simulink model "RobotArm_ForwardDynamics"  (R2024b)
settings: Solver=FixedStepAuto  StartTime=0.0  StopTime=5  FixedStep=1e-4  MaxStep=1e-4  RelTol=1e-3
InitFcn:
  | % Working Directory
  | % currDir = pwd;
  | % Import results from HoG
  | load('refAngles_HoG.mat')
  | 
  | data = thetas';
  | refA  = data(:,[1  2]);
  | refBE = data(:,[1  3]);
  | refBD = data(:,[1  4]);
  | refG  = data(:,[1  8]);
  | refH  = data(:,[1  9]);
  | refI  = data(:,[1 10]);
model workspace (MATLAB code in the model file):
  | %% General Parameters
  | 
  | g = 9.81; % [m/sec^2] assuming we are on earth :)
  | 
  | %% Chosen Parameters
  | 
  | % Gearbox Ratios
  | iA  = 20;
  | iBE = 20;
  | iBD = 20;
  | iG  = 20;
  | iH  = 20;
  | iI  = 20;
  | 
  | % Servomotor Torque Constants
  | KmA  = 0.5; % [Nm/A]
  | KmBE = 0.5; % [Nm/A]
  | KmBD = 0.5; % [Nm/A]
  | KmG  = 0.5; % [Nm/A]
  | KmH  = 0.5; % [Nm/A]
  | KmI  = 0.5; % [Nm/A]
  | 
  | %% Parameters from Project Description
  | 
  | % Servomotor Inertia for all joints
  | J_sm = 0.002; % [kg*m^2]
  | 
  | % Max Servomotor Current for all joints
  | Imax = 16; % [A]
  | 
  | % Motion Limits
  | thetaBE_max =  80; % [degrees]
  | thetaBE_min = -80; % [degrees]
  | thetaHI_max =  90; % [degrees]
  | thetaHI_min = -90; % [degrees]
  | 
  | % Spring Params
  | L0 = 0.750; % [m]
  | k = 100e3; % [N/m]
  | 
  | % Load Case
  | LCtolerance = 0.2; % [degrees]
  | 
  | %% Body Data from Appendix A
  | 
  | % Mass
  | mABC     = 750; % [kg]
  | mBE      = 250; % [kg]
  | mBDstick = 150; % [kg]
  | mBDblock = 500; % [kg]
  | mDF      = 50;  % [kg]
  | mEFG     = 150; % [kg]
  | mGH      = 200; % [kg]
  | mHI      = 100; % [kg]
  | mIJ      = 50;  % [kg]
  | 
  | % Mass Moment of Inertia about X-axis
  | Ix_ABC     = 50;  % [kg*m^2]
  | Ix_BE      = 1;   % [kg*m^2]
  | Ix_BDstick = 0.5; % [kg*m^2]
  | Ix_BDblock = 10;  % [kg*m^2]
  | Ix_DF      = 0.2; % [kg*m^2]
  | Ix_EFG     = 2;   % [kg*m^2]
  | Ix_GH      = 1;   % [kg*m^2]
  | Ix_HI      = 0.5; % [kg*m^2]
  | Ix_IJ      = 1;   % [kg*m^2]
  | 
  | % Mass Moment of Inertia about Y-axis
  | Iy_ABC     = 50; % [kg*m^2]
  | Iy_BE      = 20; % [kg*m^2]
  | Iy_BDstick = 8;  % [kg*m^2]
  | Iy_BDblock = 10; % [kg*m^2]
  | Iy_DF      = 1;  % [kg*m^2]
  | Iy_EFG     = 3;  % [kg*m^2]
  | Iy_GH      = 18; % [kg*m^2]
  | Iy_HI      = 2;  % [kg*m^2]
  | Iy_IJ      = 1;  % [kg*m^2]
  | 
  | % Mass Moment of Inertia about Z-axis
  | Iz_ABC     = 50; % [kg*m^2]
  | Iz_BE      = 20; % [kg*m^2]
  | Iz_BDstick = 8;  % [kg*m^2]
  | Iz_BDblock = 10; % [kg*m^2]
  | Iz_DF      = 1;  % [kg*m^2]
  | Iz_EFG     = 2;  % [kg*m^2]
  | Iz_GH      = 18; % [kg*m^2]
  | Iz_HI      = 2;  % [kg*m^2]
  | Iz_IJ      = 1;  % [kg*m^2]
  | 
  | %% Constant point distances
  | 
  | % Torquoise Block
  | EG = 0.225; % [m]
  | 
  | % End Effector
  | IJ_z = 0.248; % [m]
  | IJ_x = 0.235; % [m]
  | 
  | 
  | %% Geometry of Bodies
  | 
  | % All parameters which are not given
  | % are estimated from the figure
  | 
  | % Body AB - Blue Base
  | ABblock_L = 0.800; % [m]
  | ABblock_w = 2*0.240; % [m]
  | % Body BC - Blue Base Stick
  | BC_L = 0.300;  % [m]
  | BC_w = BC_L/4; % [m] NOT GIVEN, base for all sticks
  | 
  | % Body BE - Red Stick
  | BE_L = 1.050; % [m]
  | BE_w = BC_w*1.2;  % [m] NOT GIVEN
  | 
  | % Body BD - Green Block
  | BDblock_L = 0.300; % [m]
  | BDblock_w = BDblock_L; % [m] NOT GIVEN
  | % Body BD - Green Stick
  | BDstick_L = 0.800; % [m]
  | BDstick_w = BC_w;  % [m]
  | 
  | BD = 0.400; % [m]
  | 
  | % Body DF - White Stick
  | DF_L = 1.050; % [m]
  | DF_w = BC_w;  % [m]
  | 
  | % Body EFG - Torquoise block
  | EFG_L = 0.400;         % [m]
  | EFG_w = (3.5/6)*EFG_L; % [m] NOT GIVEN
  | 
  | % Body GH - Gray Stick
  | GH_L = 1.175; % [m]
  | GH_w = BC_w;  % [m] NOT GIVEN
  | 
  | % Body HI - Black Stick
  | HI_L = 0.200; % [m]
  | HI_w = BC_w;  % [m] NOT GIVEN
  | 
  | % Body IJ - (Sky Blue) End Effector Block
  | IJblock_L = (5/3.5)*IJ_x; % [m] NOT GIVEN
  | IJblock_w = (4.2/5.6)*IJ_z; % [m] NOT GIVEN
  | 
  | %% Open Loop Kinematic Parameters
  | 
  | L1 = 0.240; % [m]
  | L2 = 0.800; % [m]
  | L3 = 1.050; % [m]
  | L4 = 1.175; % [m]
  | L5 = 0.225; % [m]
  | L6 = 0.200; % [m]
  | L7 = 0.235; % [m]
  | L8 = 0.248; % [m]
  | 
  | %% Joint Visualization
  | 
  | mJ = 0.0001; % [kg]
  | 
  | % For Arms
  | r_bRJ = 0.6*BC_w; % [m]
  | l_bRJ = 2.5*BC_w; % [m]
  | r_wRJ = 0.5*BC_w; % [m]
  | l_wRJ = 2.8*BC_w; % [m]
  | 
  | % For Base
  | rB_bRJ = r_bRJ;  % [m]
  | lB_bRJ = 1.01*(ABblock_w+2*BDstick_w); % [m]
  | rB_wRJ = r_wRJ;  % [m]
  | lB_wRJ = 1.05*(ABblock_w+2*BDstick_w); % [m]
  | rBb_bRJ = r_bRJ;  % [m]
  | lBb_bRJ = 0.05*ABblock_w; % [m]
  | rBb_wRJ = r_wRJ;  % [m]
  | lBb_wRJ = 0.10*ABblock_w; % [m]
  | 
  | % r_SJ = 0.8 * w; % [m]
  | 
  | %% Point Visualization
  | 
  | P_r = 0.01; % [m]
  | 
  | %% Spring Visualization
  | 
  | spring_r = 0.05; % [m]
  | spring_L = 0.2; % [m]
  | 
  | %% Tolerances
  | 
  | maxEndEffectorAngle = 0.2; % [degrees]
undefined symbols (not defined in the file or in its folder): thetas, X, Y, Z
libraries: sm_lib x81, nesl_utility x16
(part 2 of 2)

== matlab function RobotArm_ForwardDynamics/MATLAB Function1 ==
  data: data input; A output; BD output; BE output; G output; H output; I output; t input
function [A, BD, BE, G, H, I] = splitter(data, t)

    % persistent dataLoaded
    % if isempty(dataLoaded)
    %     dataLoaded = load('refAngles_HoG.mat');
    % 
    % end
    % 
    % data = dataLoaded.thetas;
    % initialized = false;
    % if ~initialized
    %     time = data(1,:);
    %     initialized = true;
    % end

    % Extract current index
    time   = data(1,:);
    [~, idx] = min(abs(time - t));
    
    A  = data(2,idx);
    BD = data(3,idx);
    BE = data(4,idx);
    G  = data(8,idx);
    H  = data(9,idx);
    I  = data(10,idx);

end
